simulink model "Controller_First_Test"  (R2019b)
settings: Solver=VariableStepAuto  StartTime=0.0  StopTime=1000  RelTol=1e-3
values from neighbouring files (symbols this model uses):
  A = linsys.A    [Cont_ActiveSuspension.m]    (also in Cont_Hinf_Loopshaping.m; Controller1.m; X_Controller_Comparison.m; bb_mat_new.mat = [0.00600597292109 -0.00597348132103 0.0468932116793 0.001177)
  B = linsys.B    [Cont_ActiveSuspension.m]    (also in Cont_Hinf_Loopshaping.m; Controller1.m; X_Controller_Comparison.m; bb_mat_new.mat = [1.72986072315e-05  -2.70380061319e-06; -3.59799538885e-05  )
  C = linsys.C    [Cont_ActiveSuspension.m]    (also in Cont_Hinf_Loopshaping.m; Controller1.m; X_Controller_Comparison.m; bb_mat_new.mat = [-208.538516568  21.8459458344  4.23427313033  2.81126237653)
  D = linsys.D    [Cont_ActiveSuspension.m]    (also in Cont_Hinf_Loopshaping.m; Controller1.m; X_Controller_Comparison.m; bb_mat_new.mat = [0  0; 0  0])
settings Model: Creator=Presentatie  LastModifiedBy=Presentatie

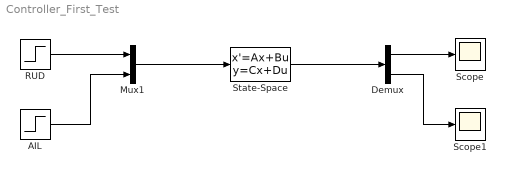
== system Controller_First_Test ==
  "AIL " : Step  SampleTime=0
  Demux : Demux  Outputs=2
  Mux1 : Mux  Inputs=2
  "RUD " : Step  SampleTime=0
  Scope : Scope
  Scope1 : Scope
  State-Space : StateSpace  A=A  B=B  C=C  D=D  InitialCondition=[0.5; 0.5; 0.5; 0.5]
  wires:
  Mux1/1 -> State-Space/1
  State-Space/1 -> Demux/1
  Demux/1 -> Scope/1
  Demux/2 -> Scope1/1
  "RUD "/1 -> Mux1/1
  "AIL "/1 -> Mux1/2
